simulink subsystem "NoElectrical"  (R2024a)
settings: Solver=VariableStepAuto  StartTime=0.0  StopTime=10.0  RelTol=1e-3
undefined symbols (not defined in the file): EnvAirTemp
settings Model: ModifiedByFormat=The MathWorks, Inc.  Creator=The MathWorks, Inc.  LastModifiedBy=The MathWorks, Inc.
settings RTWCC: GPUComputeCapability=3.5

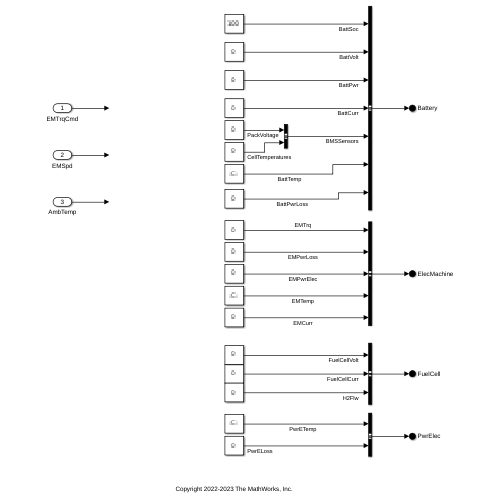
[thumbnail: Simulink's stored preview of the top-level diagram]
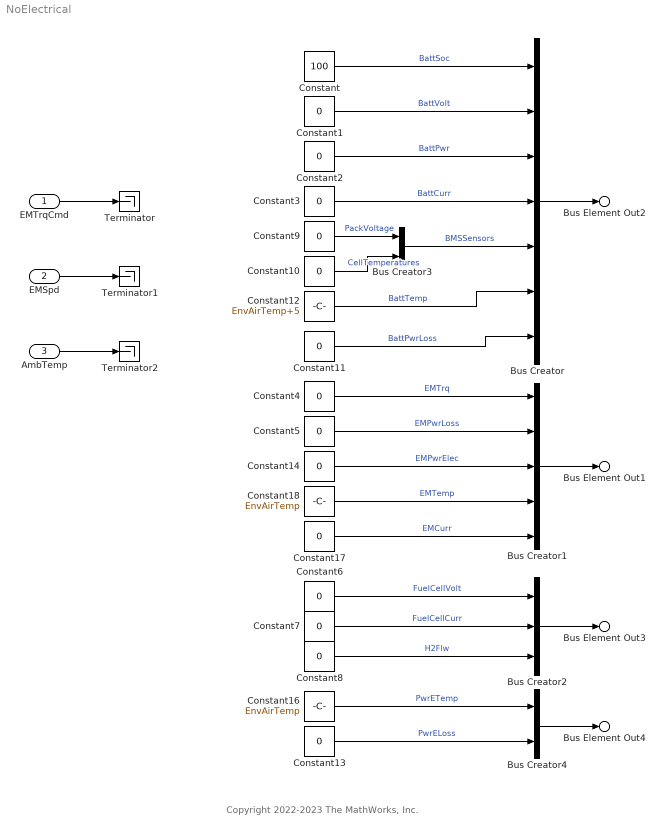
== system NoElectrical ==
  note: Copyright 2022-2023 The MathWorks, Inc.
  EMTrqCmd : Inport
  EMSpd : Inport  Port=2
  AmbTemp : Inport  Port=3
  Bus Creator : BusCreator  Inputs=7
  Bus Creator1 : BusCreator  Inputs=5
  Bus Creator2 : BusCreator  Inputs=3
  Bus Creator3 : BusCreator  Inputs=2
  Bus Creator4 : BusCreator  Inputs=2
  Constant : Constant  Value=100  SampleTime=-1
  Constant{1..11,13..14,17} (14 alike) : Constant  Value=0  SampleTime=-1
  Constant12 : Constant  Value=EnvAirTemp+5  SampleTime=-1
  Constant16 : Constant  Value=EnvAirTemp  SampleTime=-1
  Constant18 : Constant  Value=EnvAirTemp  SampleTime=-1
  Terminator : Terminator
  Terminator1 : Terminator
  Terminator2 : Terminator
  Bus Element Out2 : Outport  PortName=Battery
  Bus Element Out1 : Outport  Port=2  PortName=ElecMachine
  Bus Element Out3 : Outport  Port=3  PortName=FuelCell
  Bus Element Out4 : Outport  Port=4  PortName=PwrElec
  wires:
  Constant5/1 -> Bus Creator1/2  "EMPwrLoss"
  Bus Creator2/1 -> Bus Element Out3/1
  Bus Creator1/1 -> Bus Element Out1/1
  Bus Creator/1 -> Bus Element Out2/1
  Constant1/1 -> Bus Creator/2  "BattVolt"
  Constant/1 -> Bus Creator/1  "BattSoc"
  Constant6/1 -> Bus Creator2/1  "FuelCellVolt"
  Constant7/1 -> Bus Creator2/2  "FuelCellCurr"
  Constant3/1 -> Bus Creator/4  "BattCurr"
  Constant4/1 -> Bus Creator1/1  "EMTrq"
  EMSpd/1 -> Terminator1/1
  AmbTemp/1 -> Terminator2/1
  Constant8/1 -> Bus Creator2/3  "H2Flw"
  EMTrqCmd/1 -> Terminator/1
  Constant2/1 -> Bus Creator/3  "BattPwr"
  Bus Creator3/1 -> Bus Creator/5  "BMSSensors"
  Constant9/1 -> Bus Creator3/1  "PackVoltage"
  Constant10/1 -> Bus Creator3/2  "CellTemperatures"
  Constant11/1 -> Bus Creator/7  "BattPwrLoss"
  Constant12/1 -> Bus Creator/6  "BattTemp"
  Bus Creator4/1 -> Bus Element Out4/1
  Constant14/1 -> Bus Creator1/3  "EMPwrElec"
  Constant18/1 -> Bus Creator1/4  "EMTemp"
  Constant17/1 -> Bus Creator1/5  "EMCurr"
  Constant16/1 -> Bus Creator4/1  "PwrETemp"
  Constant13/1 -> Bus Creator4/2  "PwrELoss"
